simulink model "Model3F"  (R2014b)
settings: Solver=ode23tb  StartTime=0.0  StopTime=0.1  MaxStep=10e-6  RelTol=1e-3
values from neighbouring files (symbols this model uses):
  D = 50    [Parametri.m]
  R = 10    [Parametri.m]
  T = 1/f    (= 0.02)    [Parametri.m]
  Vg = 450    [Parametri.m]
undefined symbols (not defined in the file or in its folder): L
libraries: powerlib x21
settings Model: Creator=Zorana  LastModifiedBy=Zorana

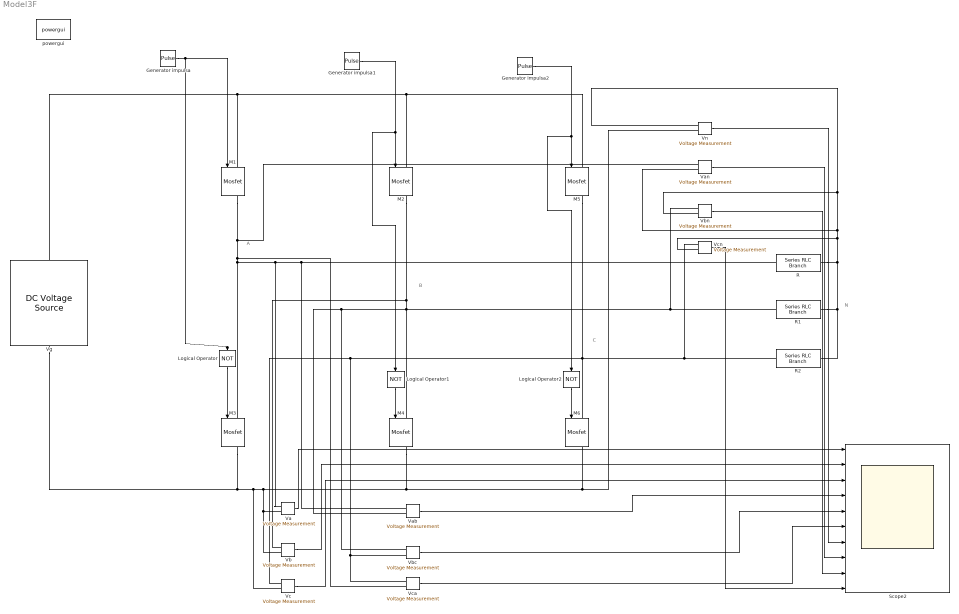
== system Model3F ==
  note: N
  note: C
  note: B
  note: A
  Generator impulsa : DiscretePulseGenerator  PulseType=Time based  Period=T  PulseWidth=D
  Generator impulsa1 : DiscretePulseGenerator  PulseType=Time based  Period=T  PulseWidth=D  PhaseDelay=T/3
  Generator impulsa2 : DiscretePulseGenerator  PulseType=Time based  Period=T  PulseWidth=D  PhaseDelay=2*T/3
  Logical Operator : Logic  Operator=NOT  IconShape=distinctive  AllPortsSameDT=off  OutDataTypeStr=boolean
  Logical Operator1 : Logic  Operator=NOT  IconShape=distinctive  AllPortsSameDT=off  OutDataTypeStr=boolean
  Logical Operator2 : Logic  Operator=NOT  IconShape=distinctive  AllPortsSameDT=off  OutDataTypeStr=boolean
  M{1..6} (6 alike) : powerlib/Power Electronics/Mosfet  Ron=1e-6  Lon=0  Rd=1e-6  Vfd=0  IC=0  Rs=1e5  Cs=inf  Measurements=on
  R : powerlib/Elements/Series RLC Branch  LConnTagsString=__new0  RConnTagsString=__new0  BranchType=R  Resistance=R  Inductance=L  SetiL0=off  InitialCurrent=0  Capacitance=1e-6  Setx0=off  InitialVoltage=0  Measurements=None
  R1 : powerlib/Elements/Series RLC Branch  LConnTagsString=__new0  RConnTagsString=__new0  BranchType=R  Resistance=R  Inductance=L  SetiL0=off  InitialCurrent=0  Capacitance=1e-6  Setx0=off  InitialVoltage=0  Measurements=None
  R2 : powerlib/Elements/Series RLC Branch  LConnTagsString=__new0  RConnTagsString=__new0  BranchType=R  Resistance=R  Inductance=L  SetiL0=off  InitialCurrent=0  Capacitance=1e-6  Setx0=off  InitialVoltage=0  Measurements=None
  Scope2 : Scope  NumInputPorts=10
      settings: YMin=-5~-5~-5~-5~-5~-5~-5~-5~-5~-5  YMax=5~5~5~5~5~5~5~5~5~5  SaveName=ScopeData2
  Va : powerlib/Measurements/Voltage Measurement  PhasorSimulation=off  OutputType=Complex  PSBequivalent=0
  Vab : powerlib/Measurements/Voltage Measurement  PhasorSimulation=off  OutputType=Complex  PSBequivalent=0
  Van : powerlib/Measurements/Voltage Measurement  PhasorSimulation=off  OutputType=Complex  PSBequivalent=0
  Vb : powerlib/Measurements/Voltage Measurement  PhasorSimulation=off  OutputType=Complex  PSBequivalent=0
  Vbc : powerlib/Measurements/Voltage Measurement  PhasorSimulation=off  OutputType=Complex  PSBequivalent=0
  Vbn : powerlib/Measurements/Voltage Measurement  PhasorSimulation=off  OutputType=Complex  PSBequivalent=0
  Vc : powerlib/Measurements/Voltage Measurement  PhasorSimulation=off  OutputType=Complex  PSBequivalent=0
  Vca : powerlib/Measurements/Voltage Measurement  PhasorSimulation=off  OutputType=Complex  PSBequivalent=0
  Vcn : powerlib/Measurements/Voltage Measurement  PhasorSimulation=off  OutputType=Complex  PSBequivalent=0
  Vg : powerlib/Electrical Sources/DC Voltage Source  Amplitude=Vg  Measurements=None
  Vn : powerlib/Measurements/Voltage Measurement  PhasorSimulation=off  OutputType=Complex  PSBequivalent=0
  powergui : powerlib/powergui  Priority=1  SimulationMode=Continuous  SolverType=Tustin/Backward Euler (TBE)  SampleTime=50e-6  frequency=60  SPID=off  DisableSnubberDevices=off  DisableRonSwitches=off  DisableVfSwitches=off  SwTol=0  DisplayEquations=off  Interpol=off  methode=off  Ts=100  frequencyindice=0  Pbase=100e6  ErrMax=1e-4  Iterations=50  UnitsV=kV  UnitsW=MW  FunctionMessages=off  echomessages=off  HookPort=off  EnableUseOfTLC=off  x0status=blocks  RestoreLinks=warning  ResistiveCurrentMeasurement=off  Frange=[0:2:500]  Ylog=off  Xlog=on  ShowGrid=off  save=off  variable=ZData  structure=0  ZoomFFT=off  StartTime=0.0  cycles=1  DisplayStyle=1  fundamental=60  FreqAxis=off  MaxFrequency=1000  frequencyindicesteady=1  RmsSteady=1  display=off
  wires:
  Generator impulsa/1 -> M1/1, Logical Operator/1
  Generator impulsa1/1 -> Logical Operator1/1, M2/1
  Generator impulsa2/1 -> Logical Operator2/1, M5/1
  Logical Operator/1 -> M3/1
  Logical Operator1/1 -> M4/1
  Logical Operator2/1 -> M6/1
  Va/1 -> Scope2/1
  Vb/1 -> Scope2/2
  Vc/1 -> Scope2/3
  Vab/1 -> Scope2/4
  Vbc/1 -> Scope2/5
  Vca/1 -> Scope2/6
  Vn/1 -> Scope2/7
  Van/1 -> Scope2/8
  Vbn/1 -> Scope2/9
  Vcn/1 -> Scope2/10
  connections:
  M1/RConn1 -- Vca/LConn2 -- Vab/LConn1 -- R/LConn1 -- Va/LConn1 -- M3/LConn1 -- Van/LConn1
  M2/RConn1 -- Vb/LConn1 -- Vbc/LConn1 -- Vab/LConn2 -- M4/LConn1 -- Vbn/LConn1 -- R1/LConn1
  M5/RConn1 -- Vcn/LConn1 -- R2/LConn1 -- Vca/LConn1 -- Vbc/LConn2 -- Vc/LConn1 -- M6/LConn1
  M3/RConn1 -- Vc/LConn2 -- Vb/LConn2 -- Va/LConn2 -- Vn/LConn2 -- M6/RConn1 -- M4/RConn1 -- Vg/LConn1
  M1/LConn1 -- M5/LConn1 -- M2/LConn1 -- Vg/RConn1
  R/RConn1 -- Vcn/LConn2 -- Vbn/LConn2 -- Vn/LConn1 -- Van/LConn2 -- R2/RConn1 -- R1/RConn1
